simulink model "stam"  (R2025a)
settings: Solver=VariableStepAuto  StartTime=0.0  StopTime=0.01  RelTol=1e-3
settings Model: Creator=user  LastModifiedBy=user

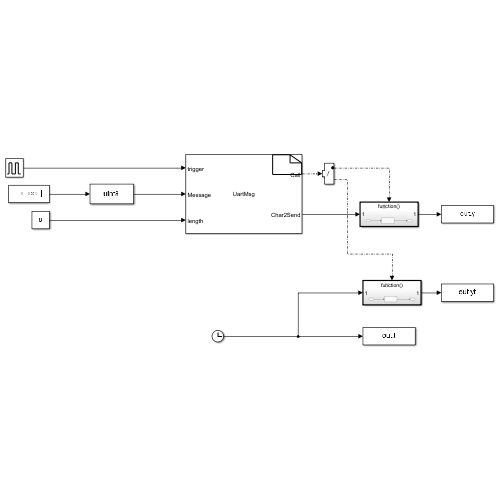
[thumbnail: Simulink's stored preview of the top-level diagram]
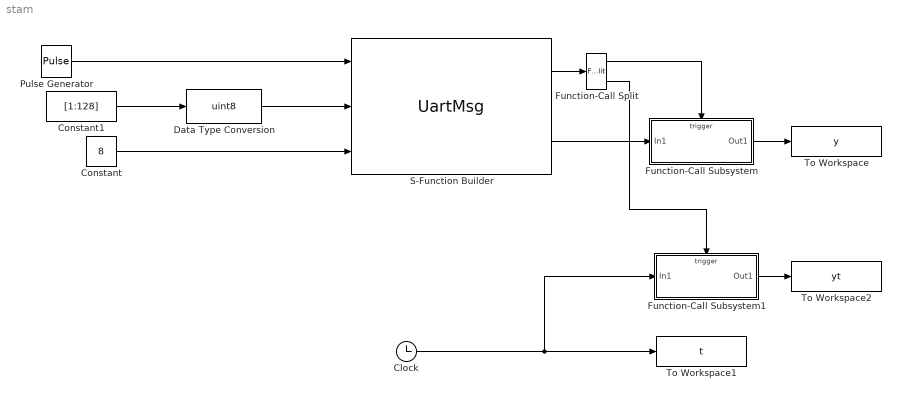
== system stam ==
  Clock : Clock
  Constant : Constant  Value=8
  Constant1 : Constant  Value=[1:128]
  Data Type Conversion : DataTypeConversion  OutDataTypeStr=uint8  SaturateOnIntegerOverflow=off  RndMeth=Floor
  Function-Call Split : FunctionCallSplit  IconShape=distinctive  NumOutputPorts=2  OutputPortLayout=default
  Function-Call Subsystem : Subsystem  TreatAsAtomicUnit=on
  Function-Call Subsystem1 : Subsystem  TreatAsAtomicUnit=on
  Pulse Generator : DiscretePulseGenerator  PulseType=Time based  Period=10  PulseWidth=5  PhaseDelay=1e-3
  S-Function Builder : S-Function  FunctionName=UartMsg  SFunctionModules=UartMsg_wrapper.c  SFunctionDeploymentMode=off  EnableBusSupport=off  mask(S-Function Builder){}
      mask help: Simulink:masks:SFunctionBuilder_MD
      mask init:
      | val = [[.9  0.75 0.75 1 1 .9 .9 1]',[1 1 0.75 0.75 .9 .9 1 .9]'];try , sys = get_param(gcb,'SfunBuilderFcnName');if isempty(sys), sys = get_param(gcb,'FunctionName'); end,catch, sys = get_param(gcb,'FunctionName'); end
      settings: CopyFcn=set_param(gcbh,'LinkStatus','none')  OpenFcn=sfunctionwizard(gcbh)
      mask Display:
      | plot(val(:,1),val(:,2))
      | disp(sys)
      | port_label('input',1,sprintf('%s', 'trigger'),'interpreter','tex')
      | port_label('input',2,sprintf('%s', 'Message'),'interpreter','tex')
      | port_label('input',3,sprintf('%s', 'length'),'interpreter','tex')
      | port_label('output',1,sprintf('%s', 'Call'),'interpreter','tex')
      | port_label('output',2,sprintf('%s', 'Char2Send'),'interpreter','tex')
  To Workspace : ToWorkspace  VariableName=y  SampleTime=1e-6
  To Workspace1 : ToWorkspace  VariableName=t  SampleTime=1e-6
  To Workspace2 : ToWorkspace  VariableName=yt  SampleTime=1e-6
  wires:
  Constant/1 -> S-Function Builder/3
  Constant1/1 -> Data Type Conversion/1
  Pulse Generator/1 -> S-Function Builder/1
  Function-Call Subsystem/1(Out1) -> To Workspace/1
  Data Type Conversion/1 -> S-Function Builder/2
  S-Function Builder/2 -> Function-Call Subsystem/1(In1)
  Clock/1 -> Function-Call Subsystem1/1(In1), To Workspace1/1
  Function-Call Subsystem1/1(Out1) -> To Workspace2/1
  S-Function Builder/1 -> Function-Call Split/1
  Function-Call Split/1 -> Function-Call Subsystem/Trigger
  Function-Call Split/2 -> Function-Call Subsystem1/Trigger

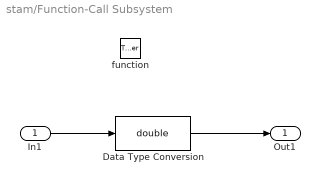
== system stam/Function-Call Subsystem ==
  In1 : Inport
  function : TriggerPort  TriggerType=function-call  VariantControl=(inherit)
  Data Type Conversion : DataTypeConversion  OutDataTypeStr=double  SaturateOnIntegerOverflow=off  RndMeth=Floor
  Out1 : Outport
  wires:
  In1/1 -> Data Type Conversion/1
  Data Type Conversion/1 -> Out1/1

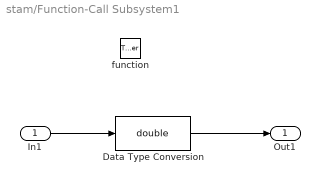
== system stam/Function-Call Subsystem1 ==
  In1 : Inport
  function : TriggerPort  TriggerType=function-call  VariantControl=(inherit)
  Data Type Conversion : DataTypeConversion  OutDataTypeStr=double  SaturateOnIntegerOverflow=off  RndMeth=Floor
  Out1 : Outport
  wires:
  In1/1 -> Data Type Conversion/1
  Data Type Conversion/1 -> Out1/1
